simulink model "Improved_Network_Model"  (R2023b)
settings: Solver=FixedStepAuto  StartTime=0.0  StopTime=0.25  FixedStep=h  RelTol=1e-3
values from neighbouring files (symbols this model uses):
  C2 = [ ... (first row only)    [Improved_Network_Constants.m]
  C3 = [ ... (first row only)    [Improved_Network_Constants.m]
  E_e = 0    [Improved_Network_Constants.m]    (also in LIF_Neuron_Constants.m)
  E_i = -70    [Improved_Network_Constants.m]    (also in LIF_Neuron_Constants.m)
  g_lut = g(lut_indices)*1000    [Improved_Network_Constants.m]    (also in LIF_Neuron_Constants.m)
  g_perceptron = 30    [Improved_Network_Constants.m]
  h = 0.0001    [Improved_Network_Constants.m]    (also in LIF_Neuron_Constants.m)
  Rm = 20*10^-2    (= 0.2)    [Improved_Network_Constants.m]    (also in LIF_Neuron_Constants.m)
  tao_m = 50*10^-3    (= 0.05)    [Improved_Network_Constants.m]    (also in LIF_Neuron_Constants.m)
  thr_val = 0.025*1000    (= 25)    [Improved_Network_Constants.m]
  V_thr = -50    [Improved_Network_Constants.m]    (also in LIF_Neuron_Constants.m)
  Vo = -65    [Improved_Network_Constants.m]    (also in LIF_Neuron_Constants.m)
libraries: hdlsllib x168
(part 1 of 4)
settings Model: Creator=Sertan  LastModifiedBy=Sertan
settings OptimizationCC: BlockReduction=off  ConditionallyExecuteInputs=off

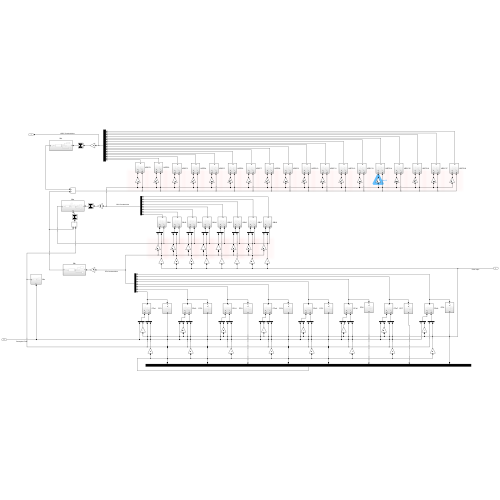
[thumbnail: Simulink's stored preview of the top-level diagram]
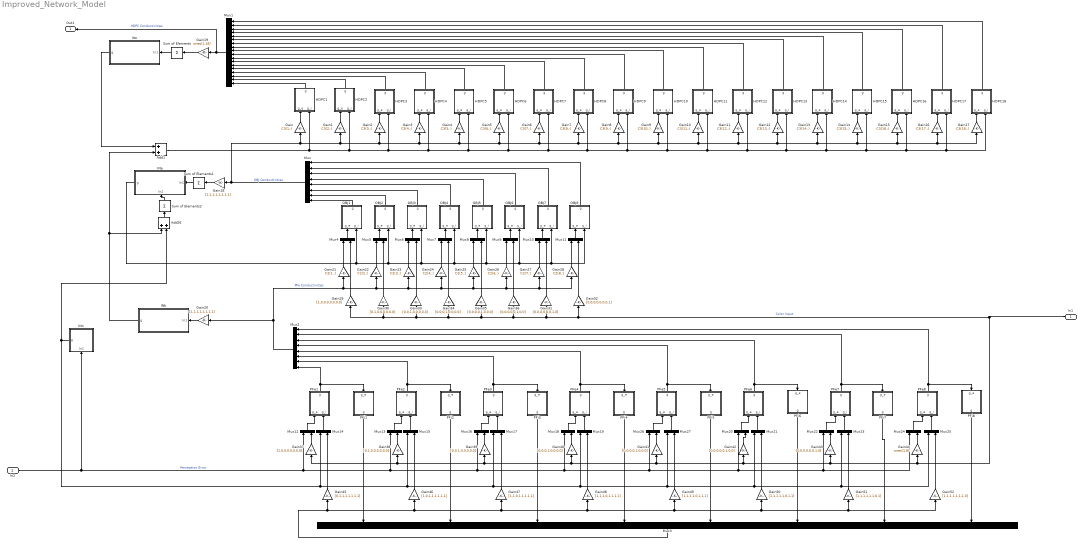
== system Improved_Network_Model ==
  In1 : Inport
  In2 : Inport  Port=2
  Add1 : Sum
  Add26 : Sum
  Gain : Gain  Gain=C3(1,:)
  Gain1 : Gain  Gain=C3(2,:)
  Gain10 : Gain  Gain=C3(11,:)
  Gain11 : Gain  Gain=C3(12,:)
  Gain12 : Gain  Gain=C3(13,:)
  Gain13 : Gain  Gain=C3(14,:)
  Gain14 : Gain  Gain=C3(15,:)
  Gain15 : Gain  Gain=C3(16,:)
  Gain16 : Gain  Gain=C3(17,:)
  Gain17 : Gain  Gain=C3(18,:)
  Gain18 : Gain  Gain=[1,1,1,1,1,1,1,1]
  Gain19 : Gain  Gain=ones(1,18)
  Gain2 : Gain  Gain=C3(3,:)
  Gain20 : Gain  Gain=[1,1,1,1,1,1,1,1]
  Gain21 : Gain  Gain=C2(1,:)  OutDataTypeStr=fixdt(1,16,8)
  Gain22 : Gain  Gain=C2(2,:)  OutDataTypeStr=fixdt(1,16,8)
  Gain23 : Gain  Gain=C2(3,:)  OutDataTypeStr=fixdt(1,16,8)
  Gain24 : Gain  Gain=C2(4,:)  OutDataTypeStr=fixdt(1,16,8)
  Gain25 : Gain  Gain=C2(5,:)  OutDataTypeStr=fixdt(1,16,8)
  Gain26 : Gain  Gain=C2(6,:)  OutDataTypeStr=fixdt(1,16,8)
  Gain27 : Gain  Gain=C2(7,:)  OutDataTypeStr=fixdt(1,16,8)
  Gain28 : Gain  Gain=C2(8,:)  OutDataTypeStr=fixdt(1,16,8)
  Gain29 : Gain  Gain=[1,0,0,0,0,0,0,0]  OutDataTypeStr=fixdt(1,16,8)
  Gain3 : Gain  Gain=C3(4,:)
  Gain30 : Gain  Gain=[0,1,0,0,0,0,0,0]  OutDataTypeStr=fixdt(1,16,8)
  Gain31 : Gain  Gain=[0,0,0,0,0,0,1,0]  OutDataTypeStr=fixdt(1,16,8)
  Gain32 : Gain  Gain=[0,0,0,0,0,0,0,1]  OutDataTypeStr=fixdt(1,16,8)
  Gain33 : Gain  Gain=[0,0,1,0,0,0,0,0]  OutDataTypeStr=fixdt(1,16,8)
  Gain34 : Gain  Gain=[0,0,0,1,0,0,0,0]  OutDataTypeStr=fixdt(1,16,8)
  Gain35 : Gain  Gain=[0,0,0,0,1,0,0,0]  OutDataTypeStr=fixdt(1,16,8)
  Gain36 : Gain  Gain=[0,0,0,0,0,1,0,0]  OutDataTypeStr=fixdt(1,16,8)
  Gain37 : Gain  Gain=[1,0,0,0,0,0,0,0]  OutDataTypeStr=fixdt(1,16,8)
  Gain38 : Gain  Gain=[0,1,0,0,0,0,0,0]  OutDataTypeStr=fixdt(1,16,8)
  Gain39 : Gain  Gain=[0,0,1,0,0,0,0,0]  OutDataTypeStr=fixdt(1,16,8)
  Gain4 : Gain  Gain=C3(5,:)
  Gain40 : Gain  Gain=[0,0,0,1,0,0,0,0]  OutDataTypeStr=fixdt(1,16,8)
  Gain41 : Gain  Gain=[0,0,0,0,1,0,0,0]  OutDataTypeStr=fixdt(1,16,8)
  Gain42 : Gain  Gain=[0,0,0,0,0,1,0,0]  OutDataTypeStr=fixdt(1,16,8)
  Gain43 : Gain  Gain=[0,0,0,0,0,0,1,0]  ParamDataTypeStr=fixdt(1,32,16)  OutDataTypeStr=fixdt(1,16,8)
  Gain44 : Gain  Gain=ones(1,8)  OutDataTypeStr=fixdt(1,16,8)
  Gain45 : Gain  Gain=[0,1,1,1,1,1,1,1]  OutDataTypeStr=fixdt(1,16,8)
  Gain46 : Gain  Gain=[1,0,1,1,1,1,1,1]  OutDataTypeStr=fixdt(1,16,8)
  Gain47 : Gain  Gain=[1,1,0,1,1,1,1,1]  OutDataTypeStr=fixdt(1,16,8)
  Gain48 : Gain  Gain=[1,1,1,0,1,1,1,1]  OutDataTypeStr=fixdt(1,16,8)
  Gain49 : Gain  Gain=[1,1,1,1,0,1,1,1]  OutDataTypeStr=fixdt(1,16,8)
  Gain5 : Gain  Gain=C3(6,:)
  Gain50 : Gain  Gain=[1,1,1,1,1,0,1,1]  OutDataTypeStr=fixdt(1,16,8)
  Gain51 : Gain  Gain=[1,1,1,1,1,1,0,1]  OutDataTypeStr=fixdt(1,16,8)
  Gain52 : Gain  Gain=[1,1,1,1,1,1,1,0]  OutDataTypeStr=fixdt(1,16,8)
  Gain6 : Gain  Gain=C3(7,:)
  Gain7 : Gain  Gain=C3(8,:)
  Gain8 : Gain  Gain=C3(9,:)
  Gain9 : Gain  Gain=C3(10,:)
  HDPC1 : Subsystem
  HDPC10 : Subsystem
  HDPC11 : Subsystem
  HDPC12 : Subsystem
  HDPC13 : Subsystem
  HDPC14 : Subsystem
  HDPC15 : Subsystem
  HDPC16 : Subsystem
  HDPC17 : Subsystem
  HDPC18 : Subsystem
  HDPC2 : Subsystem
  HDPC3 : Subsystem
  HDPC4 : Subsystem
  HDPC5 : Subsystem
  HDPC6 : Subsystem
  HDPC7 : Subsystem
  HDPC8 : Subsystem
  HDPC9 : Subsystem
  INa : Subsystem
      settings: PortSchema="{\"entries\":[{\"content\":{\"sides\":[{\"content\":{\"connectorIds\":[\"In1\"]},\"type\":\"ConnectorPlacement.EquallySpacedRectSide\",\"uuid\":\"7e874ced-1574-4e6e-b75d-ef8740d97bf8\"},{\"content\":{\"connectorIds\":[\"Out1\"],\"side\":\"RIGHT\"},\"type\":\"ConnectorPlacement.EquallySpacedRectSide\",\"uuid\":\"781db9f9-39a3-4cb8-9a9c-5cad13acfbb4\"},{\"content\":{\"side\":\"TOP\"},\"type\":\"ConnectorPlacement.EquallySpacedRectSide\",\"uuid\":\"b182c645-5fec-4e91-86bd-624479001a7a\"},{\"content\":{\"connectorIds\":[\"In2\"],\"side\":\"BOTTOM\"},\"type\":\"ConnectorPlacement.EquallySpacedRectSide\",\"uuid\":\"c39e55bf-3b54-49b1-917e-db485b5d9212\"}]},\"type\":\"ConnectorPlacement.EquallySpacedConnector\",\"uuid\":\"f02879f8-0057-4ea9-bcb0-772f9141270a\"}],\"packageUris\":[\"http://schema.mathworks.com/mf0/Connector/R2020b\"],\"version\":\"1.0\"}"
  INb : Subsystem
  INc : Subsystem
  INn : Subsystem
      settings: PortSchema="{\"entries\":[{\"content\":{\"sides\":[{\"content\":{\"connectorIds\":[\"In1\"]},\"type\":\"ConnectorPlacement.EquallySpacedRectSide\",\"uuid\":\"16d38d29-5ee4-46f0-892f-65d89b640e16\"},{\"content\":{\"side\":\"RIGHT\"},\"type\":\"ConnectorPlacement.EquallySpacedRectSide\",\"uuid\":\"2f107388-f164-4d1d-afe7-0d6d6d47ba29\"},{\"content\":{\"connectorIds\":[\"Out1\"],\"side\":\"TOP\"},\"type\":\"ConnectorPlacement.EquallySpacedRectSide\",\"uuid\":\"02c06e1d-6f05-4188-9ebd-2b49cc778128\"}]},\"type\":\"ConnectorPlacement.EquallySpacedConnector\",\"uuid\":\"ccc7dd7f-c11f-40be-8119-2d95a0a91fe7\"}],\"packageUris\":[\"http://schema.mathworks.com/mf0/Connector/R2020b\"],\"version\":\"1.0\"}"
  Mux : Mux  Inputs=8
  Mux1 : Mux  Inputs=18
  Mux{4..27} (24 alike) : Mux  Inputs=2
  Mux2 : Mux  Inputs=8
  Mux3 : Mux  Inputs=8
  OBJ1 : Subsystem
  OBJ2 : Subsystem
  OBJ3 : Subsystem
  OBJ4 : Subsystem
  OBJ5 : Subsystem
  OBJ6 : Subsystem
  OBJ7 : Subsystem
  OBJ8 : Subsystem
  PFe1 : Subsystem
  PFe2 : Subsystem
  PFe3 : Subsystem
  PFe4 : Subsystem
  PFe5 : Subsystem
  PFe6 : Subsystem
  PFe7 : Subsystem
  PFe8 : Subsystem
  PFi1 : Subsystem
  PFi2 : Subsystem
  PFi3 : Subsystem
  PFi4 : Subsystem
  PFi5 : Subsystem
  PFi6 : Subsystem
  PFi7 : Subsystem
  PFi8 : Subsystem
  Sum of Elements : Sum  Inputs=+
  Sum of Elements1 : Sum  Inputs=+
  Sum of Elements2 : Sum  Inputs=+
  Out1 : Outport  VectorParamsAs1DForOutWhenUnconnected=off
  wires:
  PFe1/1(g) -> PFi1/1(g_e), Mux2/8
  Gain5/1 -> HDPC6/1(g_e)
  Gain33/1 -> Mux6/2
  Gain44/1 -> Mux24/2
  Gain21/1 -> Mux4/1
  Gain/1 -> HDPC1/1(g_e)
  Gain31/1 -> Mux10/2
  PFi7/1(g) -> Mux3/7
  Gain29/1 -> Mux4/2
  Gain20/1 -> INb/1(In1)
  Mux21/1 -> PFe6/2(g_i)
  Gain23/1 -> Mux6/1
  Add26/1 -> Sum of Elements2/1
  HDPC6/1(g) -> Mux1/13
  Mux20/1 -> PFe6/1(g_e)
  Gain7/1 -> HDPC8/1(g_e)
  Mux24/1 -> PFe8/1(g_e)
  Gain6/1 -> HDPC7/1(g_e)
  Gain34/1 -> Mux7/2
  Gain39/1 -> Mux16/2
  Gain42/1 -> Mux20/2
  HDPC14/1(g) -> Mux1/5
  HDPC8/1(g) -> Mux1/11
  Sum of Elements/1 -> INc/1(In1)
  Mux5/1 -> OBJ2/1(g_e)
  Gain27/1 -> Mux10/1
  HDPC17/1(g) -> Mux1/2
  Gain46/1 -> Mux15/2
  Mux13/1 -> PFe2/1(g_e)
  Gain24/1 -> Mux7/1
  Gain32/1 -> Mux11/2
  Mux19/1 -> PFe4/2(g_i)
  Gain19/1 -> Sum of Elements/1
  Gain3/1 -> HDPC4/1(g_e)
  Gain35/1 -> Mux8/2
  Gain47/1 -> Mux17/2
  PFi2/1(g) -> Mux3/2
  HDPC1/1(g) -> Mux1/18
  HDPC4/1(g) -> Mux1/15
  PFi6/1(g) -> Mux3/6
  Mux14/1 -> PFe1/2(g_i)
  Gain18/1 -> Sum of Elements1/1
  HDPC18/1(g) -> Mux1/1
  Gain12/1 -> HDPC13/1(g_e)
  PFe4/1(g) -> PFi4/1(g_e), Mux2/5
  Mux25/1 -> PFe8/2(g_i)
  Mux10/1 -> OBJ7/1(g_e)
  Gain15/1 -> HDPC16/1(g_e)
  Gain28/1 -> Mux11/1
  PFi3/1(g) -> Mux3/3
  INb/1(g) -> Add1/2, Add26/1
  Gain41/1 -> Mux26/2
  Mux12/1 -> PFe1/1(g_e)
  PFe7/1(g) -> PFi7/1(g_e), Mux2/2
  PFe6/1(g) -> PFi6/1(g_e), Mux2/3
  Gain4/1 -> HDPC5/1(g_e)
  PFe8/1(g) -> PFi8/1(g_e), Mux2/1
  Gain49/1 -> Mux27/2
  Gain8/1 -> HDPC9/1(g_e)
  Mux4/1 -> OBJ1/1(g_e)
  HDPC5/1(g) -> Mux1/14
  OBJ1/1(g) -> Mux/8
  PFe3/1(g) -> PFi3/1(g_e), Mux2/6
  Mux23/1 -> PFe7/2(g_i)
  In1/1 -> Gain44/1, Gain43/1, Gain41/1, Gain37/1, Gain38/1, Gain39/1, Gain40/1, Gain42/1, Gain32/1, Gain31/1, Gain36/1, Gain29/1, Gain30/1, Gain33/1, Gain34/1, Gain35/1  "Color Input"
  Gain43/1 -> Mux22/2
  Mux/1 -> Gain18/1, Gain/1, Gain1/1, Gain2/1, Gain5/1, Gain6/1, Gain7/1, Gain9/1, Gain10/1, Gain11/1, Gain12/1, Gain13/1, Gain14/1, Gain15/1, Gain16/1, Gain17/1, Gain8/1, Gain4/1, Gain3/1  "OBJ Conductivities"
  Gain45/1 -> Mux14/2
  OBJ8/1(g) -> Mux/1
  Gain10/1 -> HDPC11/1(g_e)
  PFe5/1(g) -> PFi5/1(g_e), Mux2/4
  PFi8/1(g) -> Mux3/8
  Gain14/1 -> HDPC15/1(g_e)
  Mux9/1 -> OBJ6/1(g_e)
  PFi4/1(g) -> Mux3/4
  Mux16/1 -> PFe3/1(g_e)
  HDPC7/1(g) -> Mux1/12
  Gain13/1 -> HDPC14/1(g_e)
  INa/1(g) -> OBJ1/2(g_i), OBJ2/2(g_i), OBJ3/2(g_i), OBJ4/2(g_i), OBJ5/2(g_i), OBJ6/2(g_i), OBJ8/2(g_i), OBJ7/2(g_i)
  HDPC16/1(g) -> Mux1/3
  Mux11/1 -> OBJ8/1(g_e)
  HDPC2/1(g) -> Mux1/17
  PFe2/1(g) -> PFi2/1(g_e), Mux2/7
  Gain40/1 -> Mux18/2
  Gain9/1 -> HDPC10/1(g_e)
  HDPC9/1(g) -> Mux1/10
  Gain17/1 -> HDPC18/1(g_e)
  Gain1/1 -> HDPC2/1(g_e)
  Gain50/1 -> Mux21/2
  Mux17/1 -> PFe3/2(g_i)
  Sum of Elements2/1 -> INa/2(In2)
  Gain25/1 -> Mux8/1
  HDPC15/1(g) -> Mux1/4
  Mux26/1 -> PFe5/1(g_e)
  Mux15/1 -> PFe2/2(g_i)
  HDPC3/1(g) -> Mux1/16
  Mux22/1 -> PFe7/1(g_e)
  OBJ5/1(g) -> Mux/4
  Gain36/1 -> Mux9/2
  HDPC12/1(g) -> Mux1/7
  Gain30/1 -> Mux5/2
  Gain37/1 -> Mux12/2
  OBJ3/1(g) -> Mux/6
  Mux18/1 -> PFe4/1(g_e)
  OBJ4/1(g) -> Mux/5
  HDPC11/1(g) -> Mux1/8
  OBJ2/1(g) -> Mux/7
  Mux2/1 -> Gain27/1, Gain28/1, Gain26/1, Gain25/1, Gain24/1, Gain23/1, Gain22/1, Gain21/1, Gain20/1  "PFe Conductivities"
  Mux27/1 -> PFe5/2(g_i)
  Gain48/1 -> Mux19/2
  Gain38/1 -> Mux13/2
  Mux7/1 -> OBJ4/1(g_e)
  Gain22/1 -> Mux5/1
  Mux1/1 -> Out1/1, Gain19/1  "HDPC Conductivities"
  Gain11/1 -> HDPC12/1(g_e)
  Mux8/1 -> OBJ5/1(g_e)
  Gain2/1 -> HDPC3/1(g_e)
  Gain16/1 -> HDPC17/1(g_e)
  PFi1/1(g) -> Mux3/1
  In2/1 -> Mux18/1, Mux24/1, Mux22/1, Mux20/1, Mux26/1, Mux16/1, Mux13/1, Mux12/1, INn/1(In1)  "Perception Error"
  Sum of Elements1/1 -> INa/1(In1)
  HDPC13/1(g) -> Mux1/6
  HDPC10/1(g) -> Mux1/9
  Gain51/1 -> Mux23/2
  Mux3/1 -> Gain52/1, Gain51/1, Gain50/1, Gain49/1, Gain48/1, Gain47/1, Gain46/1, Gain45/1
  Mux6/1 -> OBJ3/1(g_e)
  PFi5/1(g) -> Mux3/5
  Gain52/1 -> Mux25/2
  INn/1(g) -> Add26/2, Mux25/1, Mux23/1, Mux21/1, Mux27/1, Mux19/1, Mux17/1, Mux15/1, Mux14/1
  Gain26/1 -> Mux9/1
  INc/1(g) -> Add1/1
  OBJ7/1(g) -> Mux/2
  Add1/1 -> HDPC1/2(g_i), HDPC2/2(g_i), HDPC3/2(g_i), HDPC4/2(g_i), HDPC5/2(g_i), HDPC6/2(g_i), HDPC7/2(g_i), HDPC8/2(g_i), HDPC9/2(g_i), HDPC10/2(g_i), HDPC11/2(g_i), HDPC12/2(g_i), HDPC13/2(g_i), HDPC14/2(g_i), HDPC15/2(g_i), HDPC16/2(g_i), HDPC17/2(g_i), HDPC18/2(g_i)
  OBJ6/1(g) -> Mux/3

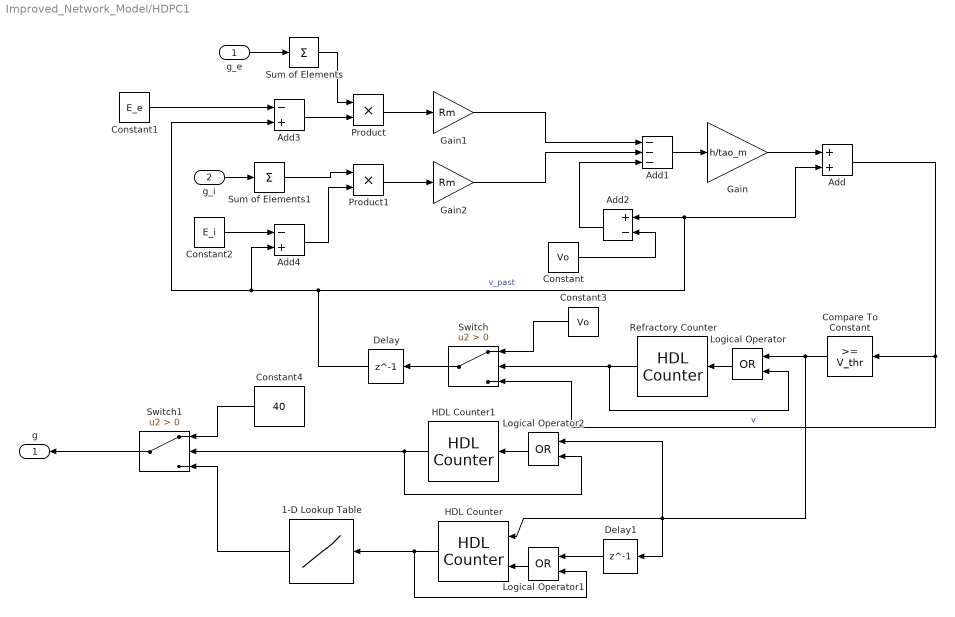
== system Improved_Network_Model/HDPC1 ==
  g_e : Inport
  g_i : Inport  Port=2
  1-D Lookup Table : Lookup_n-D  NumberOfTableDimensions=1  LookupTableObject=''  BreakpointsForDimension1=[0:201]  BreakpointsForDimension1FirstPoint=10  BreakpointsForDimension2FirstPoint=10  BreakpointsForDimension1Spacing=12  BreakpointsForDimension2Spacing=12  BreakpointsForDimension1DataTypeStr=Inherit: Inherit from 'Breakpoint data'  IndexSearchMethod=Evenly spaced points  Table=g_lut  InterpMethod=Flat  DiagnosticForOutOfRangeInput=Error  InternalRulePriority=Speed  OutDataTypeStr=fixdt(1,16,8)  RndMeth=Simplest
  Add : Sum
  Add1 : Sum  Inputs=---
  Add2 : Sum  Inputs=+-
  Add3 : Sum  Inputs=-+
  Add4 : Sum  Inputs=-+
  Compare To Constant : hdlsllib/Logic and Bit Operations/Compare To Constant  relop=>=  const=V_thr  OutDataTypeStr=boolean
  Constant : Constant  Value=Vo  OutDataTypeStr=fixdt(1,16,8)
  Constant1 : Constant  Value=E_e  OutDataTypeStr=fixdt(1,16,8)
  Constant2 : Constant  Value=E_i  OutDataTypeStr=fixdt(1,16,8)
  Constant3 : Constant  Value=Vo  OutDataTypeStr=fixdt(1,16,8)
  Constant4 : Constant  Value=40  OutDataTypeStr=fixdt(1,16,8)
  Delay : Delay  DelayLength=1  InitialCondition=Vo
  Delay1 : Delay  DelayLength=1  InitialCondition=0
  Gain : Gain  Gain=h/tao_m  OutDataTypeStr=fixdt(1,16,8)
  Gain1 : Gain  Gain=Rm
  Gain2 : Gain  Gain=Rm
  HDL Counter : hdlsllib/Sources/HDL Counter  CountType=Count limited  CountInit=0  CountStep=1  CountMax=length(g_lut)-1  CountFromType=Initial value  CountFrom=0  CountResetPort=on  CountLoadPort=off  CountEnbPort=on  CountDirPort=off  CountHitOutputPort=off  CountDataType=Unsigned  CountWordLen=8  CountFracLen=0  CountSampTime=1
  HDL Counter1 : hdlsllib/Sources/HDL Counter  CountType=Count limited  CountInit=0  CountStep=1  CountMax=2  CountFromType=Initial value  CountFrom=0  CountResetPort=off  CountLoadPort=off  CountEnbPort=on  CountDirPort=off  CountHitOutputPort=off  CountDataType=Unsigned  CountWordLen=8  CountFracLen=0  CountSampTime=1
  Logical Operator : Logic  Operator=OR  AllPortsSameDT=off  OutDataTypeStr=boolean
  Logical Operator1 : Logic  Operator=OR  AllPortsSameDT=off  OutDataTypeStr=boolean
  Logical Operator2 : Logic  Operator=OR  AllPortsSameDT=off  OutDataTypeStr=boolean
  Product : Product
  Product1 : Product
  Refractory Counter : hdlsllib/Sources/HDL Counter  CountType=Count limited  CountInit=0  CountStep=1  CountMax=r_time  CountFromType=Initial value  CountFrom=0  CountResetPort=off  CountLoadPort=off  CountEnbPort=on  CountDirPort=off  CountHitOutputPort=off  CountDataType=Unsigned  CountWordLen=8  CountFracLen=0  CountSampTime=1
  Sum of Elements : Sum  Inputs=+
  Sum of Elements1 : Sum  Inputs=+
  Switch : Switch  Criteria=u2 > Threshold  SaturateOnIntegerOverflow=off  InputSameDT=off
  Switch1 : Switch  Criteria=u2 > Threshold  OutDataTypeStr=fixdt(1,16,8)  SaturateOnIntegerOverflow=off  InputSameDT=off
  g : Outport  VectorParamsAs1DForOutWhenUnconnected=off
  wires:
  Constant/1 -> Add2/2
  Delay/1 -> Add3/2, Add4/2, Add/2, Add2/1  "v_past"
  Add/1 -> Switch/3, Compare To Constant/1  "v"
  g_i/1 -> Sum of Elements1/1
  Gain1/1 -> Add1/1
  Add2/1 -> Add1/3
  Add1/1 -> Gain/1
  Add4/1 -> Product1/2
  Product/1 -> Gain1/1
  Add3/1 -> Product/2
  Gain2/1 -> Add1/2
  Gain/1 -> Add/1
  Sum of Elements/1 -> Product/1
  Constant1/1 -> Add3/1
  Constant2/1 -> Add4/1
  Product1/1 -> Gain2/1
  Constant3/1 -> Switch/1
  Refractory Counter/1 -> Logical Operator/2, Switch/2
  Logical Operator/1 -> Refractory Counter/1
  HDL Counter/1 -> Logical Operator1/2, 1-D Lookup Table/1
  Switch1/1 -> g/1
  Switch/1 -> Delay/1
  1-D Lookup Table/1 -> Switch1/3
  Logical Operator1/1 -> HDL Counter/2
  Delay1/1 -> Logical Operator1/1
  Constant4/1 -> Switch1/1
  Logical Operator2/1 -> HDL Counter1/1
  HDL Counter1/1 -> Switch1/2, Logical Operator2/2
  Compare To Constant/1 -> Logical Operator/1, Delay1/1, Logical Operator2/1, HDL Counter/1
  g_e/1 -> Sum of Elements/1
  Sum of Elements1/1 -> Product1/1

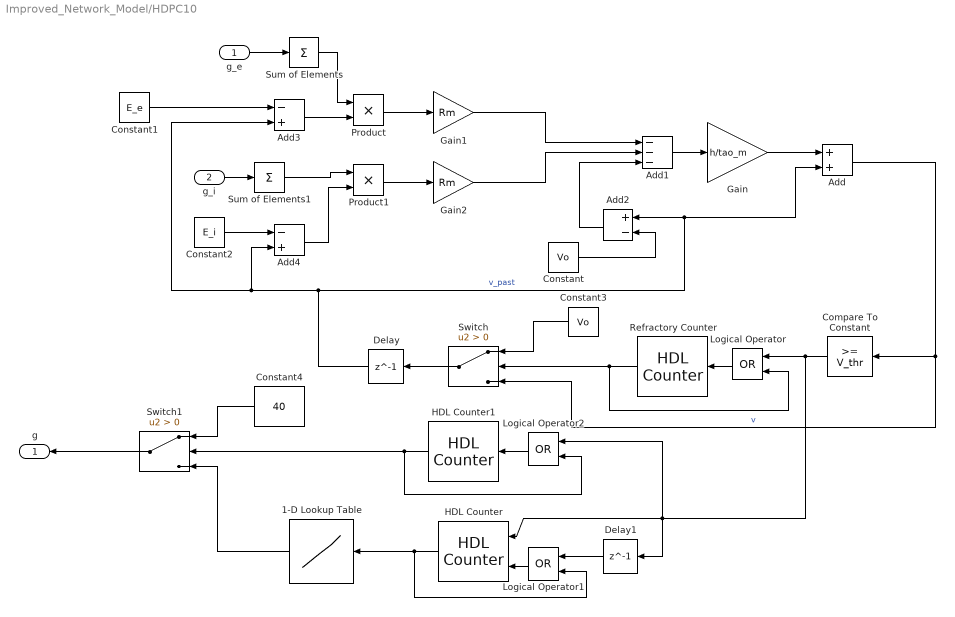
== system Improved_Network_Model/HDPC10 ==
  g_e : Inport
  g_i : Inport  Port=2
  1-D Lookup Table : Lookup_n-D  NumberOfTableDimensions=1  LookupTableObject=''  BreakpointsForDimension1=[0:201]  BreakpointsForDimension1FirstPoint=10  BreakpointsForDimension2FirstPoint=10  BreakpointsForDimension1Spacing=12  BreakpointsForDimension2Spacing=12  BreakpointsForDimension1DataTypeStr=Inherit: Inherit from 'Breakpoint data'  IndexSearchMethod=Evenly spaced points  Table=g_lut  InterpMethod=Flat  DiagnosticForOutOfRangeInput=Error  InternalRulePriority=Speed  OutDataTypeStr=fixdt(1,16,8)  RndMeth=Simplest
  Add : Sum
  Add1 : Sum  Inputs=---
  Add2 : Sum  Inputs=+-
  Add3 : Sum  Inputs=-+
  Add4 : Sum  Inputs=-+
  Compare To Constant : hdlsllib/Logic and Bit Operations/Compare To Constant  relop=>=  const=V_thr  OutDataTypeStr=boolean
  Constant : Constant  Value=Vo  OutDataTypeStr=fixdt(1,16,8)
  Constant1 : Constant  Value=E_e  OutDataTypeStr=fixdt(1,16,8)
  Constant2 : Constant  Value=E_i  OutDataTypeStr=fixdt(1,16,8)
  Constant3 : Constant  Value=Vo  OutDataTypeStr=fixdt(1,16,8)
  Constant4 : Constant  Value=40  OutDataTypeStr=fixdt(1,16,8)
  Delay : Delay  DelayLength=1  InitialCondition=Vo
  Delay1 : Delay  DelayLength=1  InitialCondition=0
  Gain : Gain  Gain=h/tao_m  OutDataTypeStr=fixdt(1,16,8)
  Gain1 : Gain  Gain=Rm
  Gain2 : Gain  Gain=Rm
  HDL Counter : hdlsllib/Sources/HDL Counter  CountType=Count limited  CountInit=0  CountStep=1  CountMax=length(g_lut)-1  CountFromType=Initial value  CountFrom=0  CountResetPort=on  CountLoadPort=off  CountEnbPort=on  CountDirPort=off  CountHitOutputPort=off  CountDataType=Unsigned  CountWordLen=8  CountFracLen=0  CountSampTime=1
  HDL Counter1 : hdlsllib/Sources/HDL Counter  CountType=Count limited  CountInit=0  CountStep=1  CountMax=2  CountFromType=Initial value  CountFrom=0  CountResetPort=off  CountLoadPort=off  CountEnbPort=on  CountDirPort=off  CountHitOutputPort=off  CountDataType=Unsigned  CountWordLen=8  CountFracLen=0  CountSampTime=1
  Logical Operator : Logic  Operator=OR  AllPortsSameDT=off  OutDataTypeStr=boolean
  Logical Operator1 : Logic  Operator=OR  AllPortsSameDT=off  OutDataTypeStr=boolean
  Logical Operator2 : Logic  Operator=OR  AllPortsSameDT=off  OutDataTypeStr=boolean
  Product : Product
  Product1 : Product
  Refractory Counter : hdlsllib/Sources/HDL Counter  CountType=Count limited  CountInit=0  CountStep=1  CountMax=r_time  CountFromType=Initial value  CountFrom=0  CountResetPort=off  CountLoadPort=off  CountEnbPort=on  CountDirPort=off  CountHitOutputPort=off  CountDataType=Unsigned  CountWordLen=8  CountFracLen=0  CountSampTime=1
  Sum of Elements : Sum  Inputs=+
  Sum of Elements1 : Sum  Inputs=+
  Switch : Switch  Criteria=u2 > Threshold  SaturateOnIntegerOverflow=off  InputSameDT=off
  Switch1 : Switch  Criteria=u2 > Threshold  OutDataTypeStr=fixdt(1,16,8)  SaturateOnIntegerOverflow=off  InputSameDT=off
  g : Outport  VectorParamsAs1DForOutWhenUnconnected=off
  wires:
  Constant/1 -> Add2/2
  Delay/1 -> Add3/2, Add4/2, Add/2, Add2/1  "v_past"
  Add/1 -> Switch/3, Compare To Constant/1  "v"
  g_i/1 -> Sum of Elements1/1
  Gain1/1 -> Add1/1
  Add2/1 -> Add1/3
  Add1/1 -> Gain/1
  Add4/1 -> Product1/2
  Product/1 -> Gain1/1
  Add3/1 -> Product/2
  Gain2/1 -> Add1/2
  Gain/1 -> Add/1
  Sum of Elements/1 -> Product/1
  Constant1/1 -> Add3/1
  Constant2/1 -> Add4/1
  Product1/1 -> Gain2/1
  Constant3/1 -> Switch/1
  Refractory Counter/1 -> Logical Operator/2, Switch/2
  Logical Operator/1 -> Refractory Counter/1
  HDL Counter/1 -> Logical Operator1/2, 1-D Lookup Table/1
  Switch1/1 -> g/1
  Switch/1 -> Delay/1
  1-D Lookup Table/1 -> Switch1/3
  Logical Operator1/1 -> HDL Counter/2
  Delay1/1 -> Logical Operator1/1
  Constant4/1 -> Switch1/1
  Logical Operator2/1 -> HDL Counter1/1
  HDL Counter1/1 -> Switch1/2, Logical Operator2/2
  Compare To Constant/1 -> Logical Operator/1, Delay1/1, Logical Operator2/1, HDL Counter/1
  g_e/1 -> Sum of Elements/1
  Sum of Elements1/1 -> Product1/1

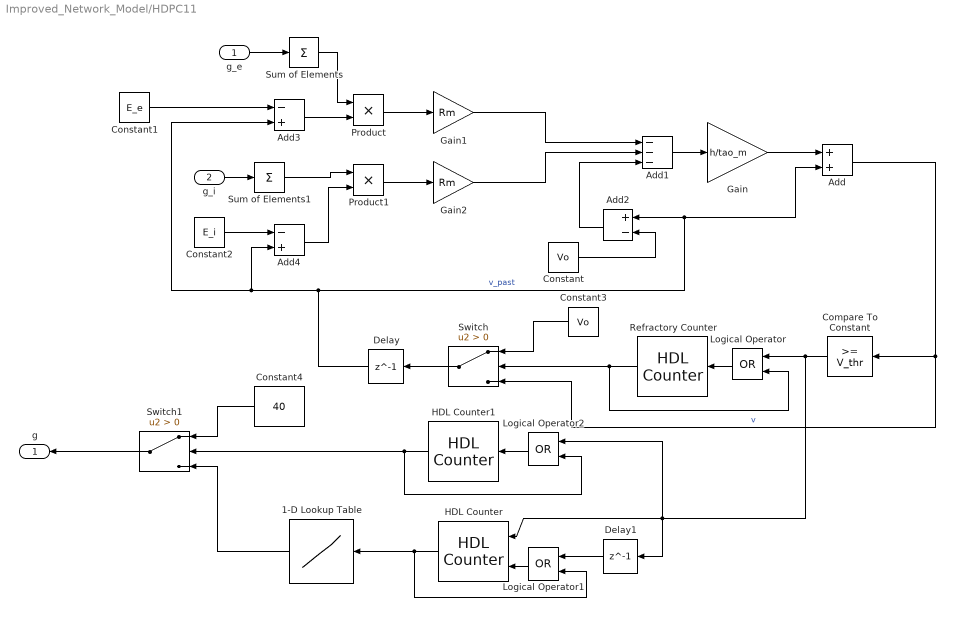
== system Improved_Network_Model/HDPC11 ==
  g_e : Inport
  g_i : Inport  Port=2
  1-D Lookup Table : Lookup_n-D  NumberOfTableDimensions=1  LookupTableObject=''  BreakpointsForDimension1=[0:201]  BreakpointsForDimension1FirstPoint=10  BreakpointsForDimension2FirstPoint=10  BreakpointsForDimension1Spacing=12  BreakpointsForDimension2Spacing=12  BreakpointsForDimension1DataTypeStr=Inherit: Inherit from 'Breakpoint data'  IndexSearchMethod=Evenly spaced points  Table=g_lut  InterpMethod=Flat  DiagnosticForOutOfRangeInput=Error  InternalRulePriority=Speed  OutDataTypeStr=fixdt(1,16,8)  RndMeth=Simplest
  Add : Sum
  Add1 : Sum  Inputs=---
  Add2 : Sum  Inputs=+-
  Add3 : Sum  Inputs=-+
  Add4 : Sum  Inputs=-+
  Compare To Constant : hdlsllib/Logic and Bit Operations/Compare To Constant  relop=>=  const=V_thr  OutDataTypeStr=boolean
  Constant : Constant  Value=Vo  OutDataTypeStr=fixdt(1,16,8)
  Constant1 : Constant  Value=E_e  OutDataTypeStr=fixdt(1,16,8)
  Constant2 : Constant  Value=E_i  OutDataTypeStr=fixdt(1,16,8)
  Constant3 : Constant  Value=Vo  OutDataTypeStr=fixdt(1,16,8)
  Constant4 : Constant  Value=40  OutDataTypeStr=fixdt(1,16,8)
  Delay : Delay  DelayLength=1  InitialCondition=Vo
  Delay1 : Delay  DelayLength=1  InitialCondition=0
  Gain : Gain  Gain=h/tao_m  OutDataTypeStr=fixdt(1,16,8)
  Gain1 : Gain  Gain=Rm
  Gain2 : Gain  Gain=Rm
  HDL Counter : hdlsllib/Sources/HDL Counter  CountType=Count limited  CountInit=0  CountStep=1  CountMax=length(g_lut)-1  CountFromType=Initial value  CountFrom=0  CountResetPort=on  CountLoadPort=off  CountEnbPort=on  CountDirPort=off  CountHitOutputPort=off  CountDataType=Unsigned  CountWordLen=8  CountFracLen=0  CountSampTime=1
  HDL Counter1 : hdlsllib/Sources/HDL Counter  CountType=Count limited  CountInit=0  CountStep=1  CountMax=2  CountFromType=Initial value  CountFrom=0  CountResetPort=off  CountLoadPort=off  CountEnbPort=on  CountDirPort=off  CountHitOutputPort=off  CountDataType=Unsigned  CountWordLen=8  CountFracLen=0  CountSampTime=1
  Logical Operator : Logic  Operator=OR  AllPortsSameDT=off  OutDataTypeStr=boolean
  Logical Operator1 : Logic  Operator=OR  AllPortsSameDT=off  OutDataTypeStr=boolean
  Logical Operator2 : Logic  Operator=OR  AllPortsSameDT=off  OutDataTypeStr=boolean
  Product : Product
  Product1 : Product
  Refractory Counter : hdlsllib/Sources/HDL Counter  CountType=Count limited  CountInit=0  CountStep=1  CountMax=r_time  CountFromType=Initial value  CountFrom=0  CountResetPort=off  CountLoadPort=off  CountEnbPort=on  CountDirPort=off  CountHitOutputPort=off  CountDataType=Unsigned  CountWordLen=8  CountFracLen=0  CountSampTime=1
  Sum of Elements : Sum  Inputs=+
  Sum of Elements1 : Sum  Inputs=+
  Switch : Switch  Criteria=u2 > Threshold  SaturateOnIntegerOverflow=off  InputSameDT=off
  Switch1 : Switch  Criteria=u2 > Threshold  OutDataTypeStr=fixdt(1,16,8)  SaturateOnIntegerOverflow=off  InputSameDT=off
  g : Outport  VectorParamsAs1DForOutWhenUnconnected=off
  wires:
  Constant/1 -> Add2/2
  Delay/1 -> Add3/2, Add4/2, Add/2, Add2/1  "v_past"
  Add/1 -> Switch/3, Compare To Constant/1  "v"
  g_i/1 -> Sum of Elements1/1
  Gain1/1 -> Add1/1
  Add2/1 -> Add1/3
  Add1/1 -> Gain/1
  Add4/1 -> Product1/2
  Product/1 -> Gain1/1
  Add3/1 -> Product/2
  Gain2/1 -> Add1/2
  Gain/1 -> Add/1
  Sum of Elements/1 -> Product/1
  Constant1/1 -> Add3/1
  Constant2/1 -> Add4/1
  Product1/1 -> Gain2/1
  Constant3/1 -> Switch/1
  Refractory Counter/1 -> Logical Operator/2, Switch/2
  Logical Operator/1 -> Refractory Counter/1
  HDL Counter/1 -> Logical Operator1/2, 1-D Lookup Table/1
  Switch1/1 -> g/1
  Switch/1 -> Delay/1
  1-D Lookup Table/1 -> Switch1/3
  Logical Operator1/1 -> HDL Counter/2
  Delay1/1 -> Logical Operator1/1
  Constant4/1 -> Switch1/1
  Logical Operator2/1 -> HDL Counter1/1
  HDL Counter1/1 -> Switch1/2, Logical Operator2/2
  Compare To Constant/1 -> Logical Operator/1, Delay1/1, Logical Operator2/1, HDL Counter/1
  g_e/1 -> Sum of Elements/1
  Sum of Elements1/1 -> Product1/1

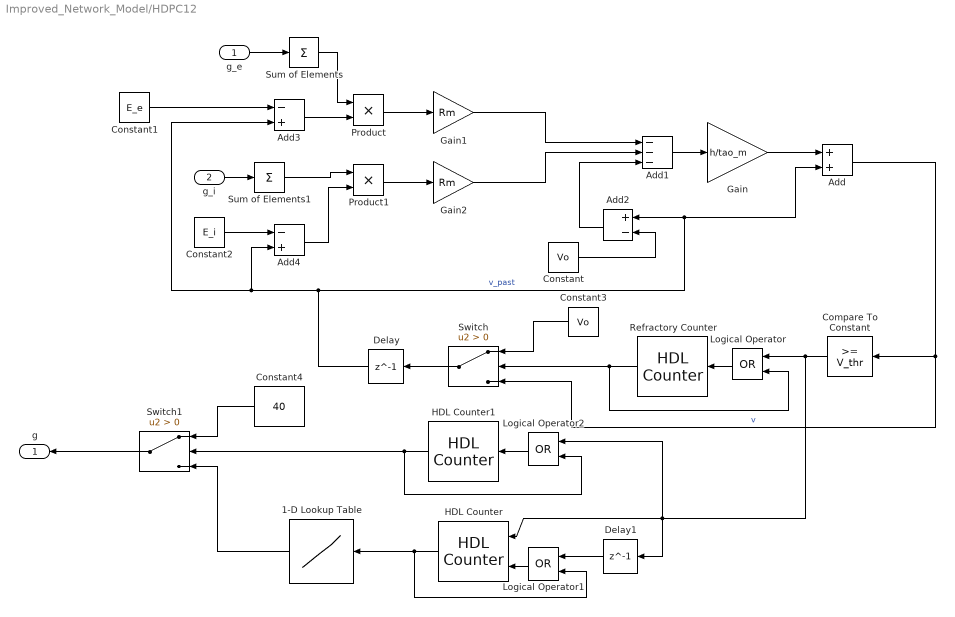
== system Improved_Network_Model/HDPC12 ==
  g_e : Inport
  g_i : Inport  Port=2
  1-D Lookup Table : Lookup_n-D  NumberOfTableDimensions=1  LookupTableObject=''  BreakpointsForDimension1=[0:201]  BreakpointsForDimension1FirstPoint=10  BreakpointsForDimension2FirstPoint=10  BreakpointsForDimension1Spacing=12  BreakpointsForDimension2Spacing=12  BreakpointsForDimension1DataTypeStr=Inherit: Inherit from 'Breakpoint data'  IndexSearchMethod=Evenly spaced points  Table=g_lut  InterpMethod=Flat  DiagnosticForOutOfRangeInput=Error  InternalRulePriority=Speed  OutDataTypeStr=fixdt(1,16,8)  RndMeth=Simplest
  Add : Sum
  Add1 : Sum  Inputs=---
  Add2 : Sum  Inputs=+-
  Add3 : Sum  Inputs=-+
  Add4 : Sum  Inputs=-+
  Compare To Constant : hdlsllib/Logic and Bit Operations/Compare To Constant  relop=>=  const=V_thr  OutDataTypeStr=boolean
  Constant : Constant  Value=Vo  OutDataTypeStr=fixdt(1,16,8)
  Constant1 : Constant  Value=E_e  OutDataTypeStr=fixdt(1,16,8)
  Constant2 : Constant  Value=E_i  OutDataTypeStr=fixdt(1,16,8)
  Constant3 : Constant  Value=Vo  OutDataTypeStr=fixdt(1,16,8)
  Constant4 : Constant  Value=40  OutDataTypeStr=fixdt(1,16,8)
  Delay : Delay  DelayLength=1  InitialCondition=Vo
  Delay1 : Delay  DelayLength=1  InitialCondition=0
  Gain : Gain  Gain=h/tao_m  OutDataTypeStr=fixdt(1,16,8)
  Gain1 : Gain  Gain=Rm
  Gain2 : Gain  Gain=Rm
  HDL Counter : hdlsllib/Sources/HDL Counter  CountType=Count limited  CountInit=0  CountStep=1  CountMax=length(g_lut)-1  CountFromType=Initial value  CountFrom=0  CountResetPort=on  CountLoadPort=off  CountEnbPort=on  CountDirPort=off  CountHitOutputPort=off  CountDataType=Unsigned  CountWordLen=8  CountFracLen=0  CountSampTime=1
  HDL Counter1 : hdlsllib/Sources/HDL Counter  CountType=Count limited  CountInit=0  CountStep=1  CountMax=2  CountFromType=Initial value  CountFrom=0  CountResetPort=off  CountLoadPort=off  CountEnbPort=on  CountDirPort=off  CountHitOutputPort=off  CountDataType=Unsigned  CountWordLen=8  CountFracLen=0  CountSampTime=1
  Logical Operator : Logic  Operator=OR  AllPortsSameDT=off  OutDataTypeStr=boolean
  Logical Operator1 : Logic  Operator=OR  AllPortsSameDT=off  OutDataTypeStr=boolean
  Logical Operator2 : Logic  Operator=OR  AllPortsSameDT=off  OutDataTypeStr=boolean
  Product : Product
  Product1 : Product
  Refractory Counter : hdlsllib/Sources/HDL Counter  CountType=Count limited  CountInit=0  CountStep=1  CountMax=r_time  CountFromType=Initial value  CountFrom=0  CountResetPort=off  CountLoadPort=off  CountEnbPort=on  CountDirPort=off  CountHitOutputPort=off  CountDataType=Unsigned  CountWordLen=8  CountFracLen=0  CountSampTime=1
  Sum of Elements : Sum  Inputs=+
  Sum of Elements1 : Sum  Inputs=+
  Switch : Switch  Criteria=u2 > Threshold  SaturateOnIntegerOverflow=off  InputSameDT=off
  Switch1 : Switch  Criteria=u2 > Threshold  OutDataTypeStr=fixdt(1,16,8)  SaturateOnIntegerOverflow=off  InputSameDT=off
  g : Outport  VectorParamsAs1DForOutWhenUnconnected=off
  wires:
  Constant/1 -> Add2/2
  Delay/1 -> Add3/2, Add4/2, Add/2, Add2/1  "v_past"
  Add/1 -> Switch/3, Compare To Constant/1  "v"
  g_i/1 -> Sum of Elements1/1
  Gain1/1 -> Add1/1
  Add2/1 -> Add1/3
  Add1/1 -> Gain/1
  Add4/1 -> Product1/2
  Product/1 -> Gain1/1
  Add3/1 -> Product/2
  Gain2/1 -> Add1/2
  Gain/1 -> Add/1
  Sum of Elements/1 -> Product/1
  Constant1/1 -> Add3/1
  Constant2/1 -> Add4/1
  Product1/1 -> Gain2/1
  Constant3/1 -> Switch/1
  Refractory Counter/1 -> Logical Operator/2, Switch/2
  Logical Operator/1 -> Refractory Counter/1
  HDL Counter/1 -> Logical Operator1/2, 1-D Lookup Table/1
  Switch1/1 -> g/1
  Switch/1 -> Delay/1
  1-D Lookup Table/1 -> Switch1/3
  Logical Operator1/1 -> HDL Counter/2
  Delay1/1 -> Logical Operator1/1
  Constant4/1 -> Switch1/1
  Logical Operator2/1 -> HDL Counter1/1
  HDL Counter1/1 -> Switch1/2, Logical Operator2/2
  Compare To Constant/1 -> Logical Operator/1, Delay1/1, Logical Operator2/1, HDL Counter/1
  g_e/1 -> Sum of Elements/1
  Sum of Elements1/1 -> Product1/1

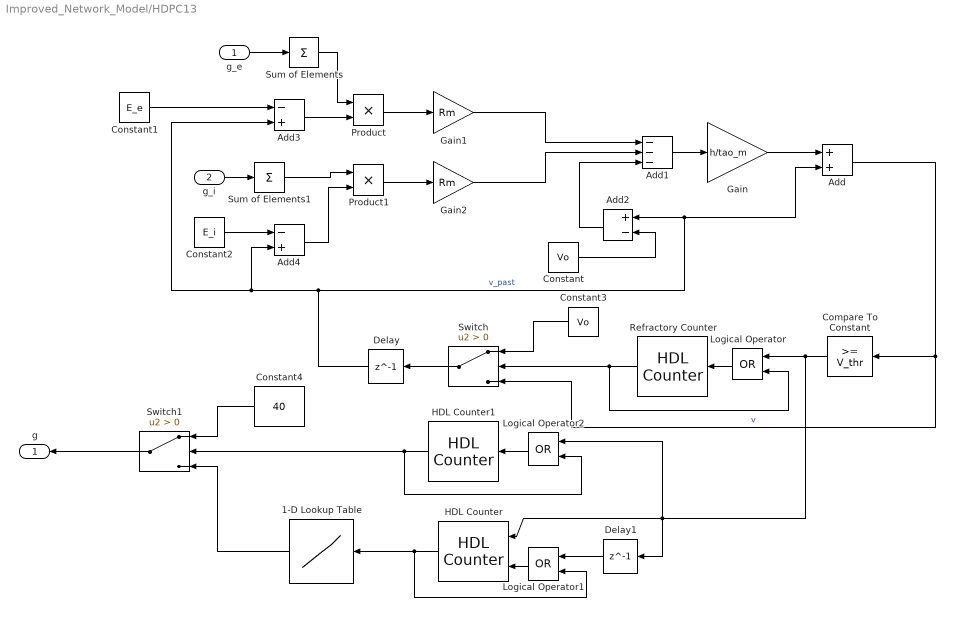
== system Improved_Network_Model/HDPC13 ==
  g_e : Inport
  g_i : Inport  Port=2
  1-D Lookup Table : Lookup_n-D  NumberOfTableDimensions=1  LookupTableObject=''  BreakpointsForDimension1=[0:201]  BreakpointsForDimension1FirstPoint=10  BreakpointsForDimension2FirstPoint=10  BreakpointsForDimension1Spacing=12  BreakpointsForDimension2Spacing=12  BreakpointsForDimension1DataTypeStr=Inherit: Inherit from 'Breakpoint data'  IndexSearchMethod=Evenly spaced points  Table=g_lut  InterpMethod=Flat  DiagnosticForOutOfRangeInput=Error  InternalRulePriority=Speed  OutDataTypeStr=fixdt(1,16,8)  RndMeth=Simplest
  Add : Sum
  Add1 : Sum  Inputs=---
  Add2 : Sum  Inputs=+-
  Add3 : Sum  Inputs=-+
  Add4 : Sum  Inputs=-+
  Compare To Constant : hdlsllib/Logic and Bit Operations/Compare To Constant  relop=>=  const=V_thr  OutDataTypeStr=boolean
  Constant : Constant  Value=Vo  OutDataTypeStr=fixdt(1,16,8)
  Constant1 : Constant  Value=E_e  OutDataTypeStr=fixdt(1,16,8)
  Constant2 : Constant  Value=E_i  OutDataTypeStr=fixdt(1,16,8)
  Constant3 : Constant  Value=Vo  OutDataTypeStr=fixdt(1,16,8)
  Constant4 : Constant  Value=40  OutDataTypeStr=fixdt(1,16,8)
  Delay : Delay  DelayLength=1  InitialCondition=Vo
  Delay1 : Delay  DelayLength=1  InitialCondition=0
  Gain : Gain  Gain=h/tao_m  OutDataTypeStr=fixdt(1,16,8)
  Gain1 : Gain  Gain=Rm
  Gain2 : Gain  Gain=Rm
  HDL Counter : hdlsllib/Sources/HDL Counter  CountType=Count limited  CountInit=0  CountStep=1  CountMax=length(g_lut)-1  CountFromType=Initial value  CountFrom=0  CountResetPort=on  CountLoadPort=off  CountEnbPort=on  CountDirPort=off  CountHitOutputPort=off  CountDataType=Unsigned  CountWordLen=8  CountFracLen=0  CountSampTime=1
  HDL Counter1 : hdlsllib/Sources/HDL Counter  CountType=Count limited  CountInit=0  CountStep=1  CountMax=2  CountFromType=Initial value  CountFrom=0  CountResetPort=off  CountLoadPort=off  CountEnbPort=on  CountDirPort=off  CountHitOutputPort=off  CountDataType=Unsigned  CountWordLen=8  CountFracLen=0  CountSampTime=1
  Logical Operator : Logic  Operator=OR  AllPortsSameDT=off  OutDataTypeStr=boolean
  Logical Operator1 : Logic  Operator=OR  AllPortsSameDT=off  OutDataTypeStr=boolean
  Logical Operator2 : Logic  Operator=OR  AllPortsSameDT=off  OutDataTypeStr=boolean
  Product : Product
  Product1 : Product
  Refractory Counter : hdlsllib/Sources/HDL Counter  CountType=Count limited  CountInit=0  CountStep=1  CountMax=r_time  CountFromType=Initial value  CountFrom=0  CountResetPort=off  CountLoadPort=off  CountEnbPort=on  CountDirPort=off  CountHitOutputPort=off  CountDataType=Unsigned  CountWordLen=8  CountFracLen=0  CountSampTime=1
  Sum of Elements : Sum  Inputs=+
  Sum of Elements1 : Sum  Inputs=+
  Switch : Switch  Criteria=u2 > Threshold  SaturateOnIntegerOverflow=off  InputSameDT=off
  Switch1 : Switch  Criteria=u2 > Threshold  OutDataTypeStr=fixdt(1,16,8)  SaturateOnIntegerOverflow=off  InputSameDT=off
  g : Outport  VectorParamsAs1DForOutWhenUnconnected=off
  wires:
  Constant/1 -> Add2/2
  Delay/1 -> Add3/2, Add4/2, Add/2, Add2/1  "v_past"
  Add/1 -> Switch/3, Compare To Constant/1  "v"
  g_i/1 -> Sum of Elements1/1
  Gain1/1 -> Add1/1
  Add2/1 -> Add1/3
  Add1/1 -> Gain/1
  Add4/1 -> Product1/2
  Product/1 -> Gain1/1
  Add3/1 -> Product/2
  Gain2/1 -> Add1/2
  Gain/1 -> Add/1
  Sum of Elements/1 -> Product/1
  Constant1/1 -> Add3/1
  Constant2/1 -> Add4/1
  Product1/1 -> Gain2/1
  Constant3/1 -> Switch/1
  Refractory Counter/1 -> Logical Operator/2, Switch/2
  Logical Operator/1 -> Refractory Counter/1
  HDL Counter/1 -> Logical Operator1/2, 1-D Lookup Table/1
  Switch1/1 -> g/1
  Switch/1 -> Delay/1
  1-D Lookup Table/1 -> Switch1/3
  Logical Operator1/1 -> HDL Counter/2
  Delay1/1 -> Logical Operator1/1
  Constant4/1 -> Switch1/1
  Logical Operator2/1 -> HDL Counter1/1
  HDL Counter1/1 -> Switch1/2, Logical Operator2/2
  Compare To Constant/1 -> Logical Operator/1, Delay1/1, Logical Operator2/1, HDL Counter/1
  g_e/1 -> Sum of Elements/1
  Sum of Elements1/1 -> Product1/1

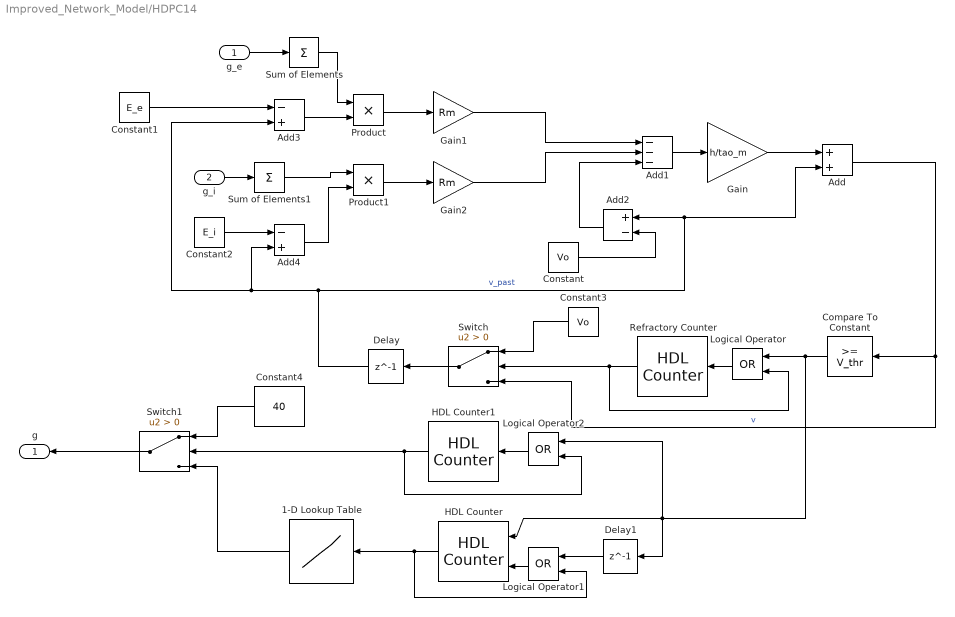
== system Improved_Network_Model/HDPC14 ==
  g_e : Inport
  g_i : Inport  Port=2
  1-D Lookup Table : Lookup_n-D  NumberOfTableDimensions=1  LookupTableObject=''  BreakpointsForDimension1=[0:201]  BreakpointsForDimension1FirstPoint=10  BreakpointsForDimension2FirstPoint=10  BreakpointsForDimension1Spacing=12  BreakpointsForDimension2Spacing=12  BreakpointsForDimension1DataTypeStr=Inherit: Inherit from 'Breakpoint data'  IndexSearchMethod=Evenly spaced points  Table=g_lut  InterpMethod=Flat  DiagnosticForOutOfRangeInput=Error  InternalRulePriority=Speed  OutDataTypeStr=fixdt(1,16,8)  RndMeth=Simplest
  Add : Sum
  Add1 : Sum  Inputs=---
  Add2 : Sum  Inputs=+-
  Add3 : Sum  Inputs=-+
  Add4 : Sum  Inputs=-+
  Compare To Constant : hdlsllib/Logic and Bit Operations/Compare To Constant  relop=>=  const=V_thr  OutDataTypeStr=boolean
  Constant : Constant  Value=Vo  OutDataTypeStr=fixdt(1,16,8)
  Constant1 : Constant  Value=E_e  OutDataTypeStr=fixdt(1,16,8)
  Constant2 : Constant  Value=E_i  OutDataTypeStr=fixdt(1,16,8)
  Constant3 : Constant  Value=Vo  OutDataTypeStr=fixdt(1,16,8)
  Constant4 : Constant  Value=40  OutDataTypeStr=fixdt(1,16,8)
  Delay : Delay  DelayLength=1  InitialCondition=Vo
  Delay1 : Delay  DelayLength=1  InitialCondition=0
  Gain : Gain  Gain=h/tao_m  OutDataTypeStr=fixdt(1,16,8)
  Gain1 : Gain  Gain=Rm
  Gain2 : Gain  Gain=Rm
  HDL Counter : hdlsllib/Sources/HDL Counter  CountType=Count limited  CountInit=0  CountStep=1  CountMax=length(g_lut)-1  CountFromType=Initial value  CountFrom=0  CountResetPort=on  CountLoadPort=off  CountEnbPort=on  CountDirPort=off  CountHitOutputPort=off  CountDataType=Unsigned  CountWordLen=8  CountFracLen=0  CountSampTime=1
  HDL Counter1 : hdlsllib/Sources/HDL Counter  CountType=Count limited  CountInit=0  CountStep=1  CountMax=2  CountFromType=Initial value  CountFrom=0  CountResetPort=off  CountLoadPort=off  CountEnbPort=on  CountDirPort=off  CountHitOutputPort=off  CountDataType=Unsigned  CountWordLen=8  CountFracLen=0  CountSampTime=1
  Logical Operator : Logic  Operator=OR  AllPortsSameDT=off  OutDataTypeStr=boolean
  Logical Operator1 : Logic  Operator=OR  AllPortsSameDT=off  OutDataTypeStr=boolean
  Logical Operator2 : Logic  Operator=OR  AllPortsSameDT=off  OutDataTypeStr=boolean
  Product : Product
  Product1 : Product
  Refractory Counter : hdlsllib/Sources/HDL Counter  CountType=Count limited  CountInit=0  CountStep=1  CountMax=r_time  CountFromType=Initial value  CountFrom=0  CountResetPort=off  CountLoadPort=off  CountEnbPort=on  CountDirPort=off  CountHitOutputPort=off  CountDataType=Unsigned  CountWordLen=8  CountFracLen=0  CountSampTime=1
  Sum of Elements : Sum  Inputs=+
  Sum of Elements1 : Sum  Inputs=+
  Switch : Switch  Criteria=u2 > Threshold  SaturateOnIntegerOverflow=off  InputSameDT=off
  Switch1 : Switch  Criteria=u2 > Threshold  OutDataTypeStr=fixdt(1,16,8)  SaturateOnIntegerOverflow=off  InputSameDT=off
  g : Outport  VectorParamsAs1DForOutWhenUnconnected=off
  wires:
  Constant/1 -> Add2/2
  Delay/1 -> Add3/2, Add4/2, Add/2, Add2/1  "v_past"
  Add/1 -> Switch/3, Compare To Constant/1  "v"
  g_i/1 -> Sum of Elements1/1
  Gain1/1 -> Add1/1
  Add2/1 -> Add1/3
  Add1/1 -> Gain/1
  Add4/1 -> Product1/2
  Product/1 -> Gain1/1
  Add3/1 -> Product/2
  Gain2/1 -> Add1/2
  Gain/1 -> Add/1
  Sum of Elements/1 -> Product/1
  Constant1/1 -> Add3/1
  Constant2/1 -> Add4/1
  Product1/1 -> Gain2/1
  Constant3/1 -> Switch/1
  Refractory Counter/1 -> Logical Operator/2, Switch/2
  Logical Operator/1 -> Refractory Counter/1
  HDL Counter/1 -> Logical Operator1/2, 1-D Lookup Table/1
  Switch1/1 -> g/1
  Switch/1 -> Delay/1
  1-D Lookup Table/1 -> Switch1/3
  Logical Operator1/1 -> HDL Counter/2
  Delay1/1 -> Logical Operator1/1
  Constant4/1 -> Switch1/1
  Logical Operator2/1 -> HDL Counter1/1
  HDL Counter1/1 -> Switch1/2, Logical Operator2/2
  Compare To Constant/1 -> Logical Operator/1, Delay1/1, Logical Operator2/1, HDL Counter/1
  g_e/1 -> Sum of Elements/1
  Sum of Elements1/1 -> Product1/1

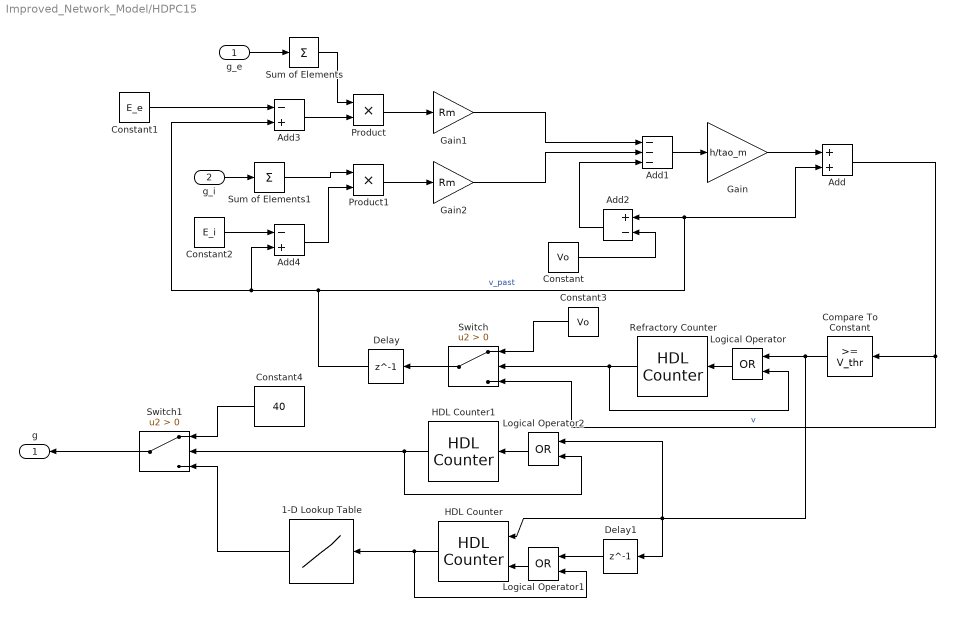
== system Improved_Network_Model/HDPC15 ==
  g_e : Inport
  g_i : Inport  Port=2
  1-D Lookup Table : Lookup_n-D  NumberOfTableDimensions=1  LookupTableObject=''  BreakpointsForDimension1=[0:201]  BreakpointsForDimension1FirstPoint=10  BreakpointsForDimension2FirstPoint=10  BreakpointsForDimension1Spacing=12  BreakpointsForDimension2Spacing=12  BreakpointsForDimension1DataTypeStr=Inherit: Inherit from 'Breakpoint data'  IndexSearchMethod=Evenly spaced points  Table=g_lut  InterpMethod=Flat  DiagnosticForOutOfRangeInput=Error  InternalRulePriority=Speed  OutDataTypeStr=fixdt(1,16,8)  RndMeth=Simplest
  Add : Sum
  Add1 : Sum  Inputs=---
  Add2 : Sum  Inputs=+-
  Add3 : Sum  Inputs=-+
  Add4 : Sum  Inputs=-+
  Compare To Constant : hdlsllib/Logic and Bit Operations/Compare To Constant  relop=>=  const=V_thr  OutDataTypeStr=boolean
  Constant : Constant  Value=Vo  OutDataTypeStr=fixdt(1,16,8)
  Constant1 : Constant  Value=E_e  OutDataTypeStr=fixdt(1,16,8)
  Constant2 : Constant  Value=E_i  OutDataTypeStr=fixdt(1,16,8)
  Constant3 : Constant  Value=Vo  OutDataTypeStr=fixdt(1,16,8)
  Constant4 : Constant  Value=40  OutDataTypeStr=fixdt(1,16,8)
  Delay : Delay  DelayLength=1  InitialCondition=Vo
  Delay1 : Delay  DelayLength=1  InitialCondition=0
  Gain : Gain  Gain=h/tao_m  OutDataTypeStr=fixdt(1,16,8)
  Gain1 : Gain  Gain=Rm
  Gain2 : Gain  Gain=Rm
  HDL Counter : hdlsllib/Sources/HDL Counter  CountType=Count limited  CountInit=0  CountStep=1  CountMax=length(g_lut)-1  CountFromType=Initial value  CountFrom=0  CountResetPort=on  CountLoadPort=off  CountEnbPort=on  CountDirPort=off  CountHitOutputPort=off  CountDataType=Unsigned  CountWordLen=8  CountFracLen=0  CountSampTime=1
  HDL Counter1 : hdlsllib/Sources/HDL Counter  CountType=Count limited  CountInit=0  CountStep=1  CountMax=2  CountFromType=Initial value  CountFrom=0  CountResetPort=off  CountLoadPort=off  CountEnbPort=on  CountDirPort=off  CountHitOutputPort=off  CountDataType=Unsigned  CountWordLen=8  CountFracLen=0  CountSampTime=1
  Logical Operator : Logic  Operator=OR  AllPortsSameDT=off  OutDataTypeStr=boolean
  Logical Operator1 : Logic  Operator=OR  AllPortsSameDT=off  OutDataTypeStr=boolean
  Logical Operator2 : Logic  Operator=OR  AllPortsSameDT=off  OutDataTypeStr=boolean
  Product : Product
  Product1 : Product
  Refractory Counter : hdlsllib/Sources/HDL Counter  CountType=Count limited  CountInit=0  CountStep=1  CountMax=r_time  CountFromType=Initial value  CountFrom=0  CountResetPort=off  CountLoadPort=off  CountEnbPort=on  CountDirPort=off  CountHitOutputPort=off  CountDataType=Unsigned  CountWordLen=8  CountFracLen=0  CountSampTime=1
  Sum of Elements : Sum  Inputs=+
  Sum of Elements1 : Sum  Inputs=+
  Switch : Switch  Criteria=u2 > Threshold  SaturateOnIntegerOverflow=off  InputSameDT=off
  Switch1 : Switch  Criteria=u2 > Threshold  OutDataTypeStr=fixdt(1,16,8)  SaturateOnIntegerOverflow=off  InputSameDT=off
  g : Outport  VectorParamsAs1DForOutWhenUnconnected=off
  wires:
  Constant/1 -> Add2/2
  Delay/1 -> Add3/2, Add4/2, Add/2, Add2/1  "v_past"
  Add/1 -> Switch/3, Compare To Constant/1  "v"
  g_i/1 -> Sum of Elements1/1
  Gain1/1 -> Add1/1
  Add2/1 -> Add1/3
  Add1/1 -> Gain/1
  Add4/1 -> Product1/2
  Product/1 -> Gain1/1
  Add3/1 -> Product/2
  Gain2/1 -> Add1/2
  Gain/1 -> Add/1
  Sum of Elements/1 -> Product/1
  Constant1/1 -> Add3/1
  Constant2/1 -> Add4/1
  Product1/1 -> Gain2/1
  Constant3/1 -> Switch/1
  Refractory Counter/1 -> Logical Operator/2, Switch/2
  Logical Operator/1 -> Refractory Counter/1
  HDL Counter/1 -> Logical Operator1/2, 1-D Lookup Table/1
  Switch1/1 -> g/1
  Switch/1 -> Delay/1
  1-D Lookup Table/1 -> Switch1/3
  Logical Operator1/1 -> HDL Counter/2
  Delay1/1 -> Logical Operator1/1
  Constant4/1 -> Switch1/1
  Logical Operator2/1 -> HDL Counter1/1
  HDL Counter1/1 -> Switch1/2, Logical Operator2/2
  Compare To Constant/1 -> Logical Operator/1, Delay1/1, Logical Operator2/1, HDL Counter/1
  g_e/1 -> Sum of Elements/1
  Sum of Elements1/1 -> Product1/1

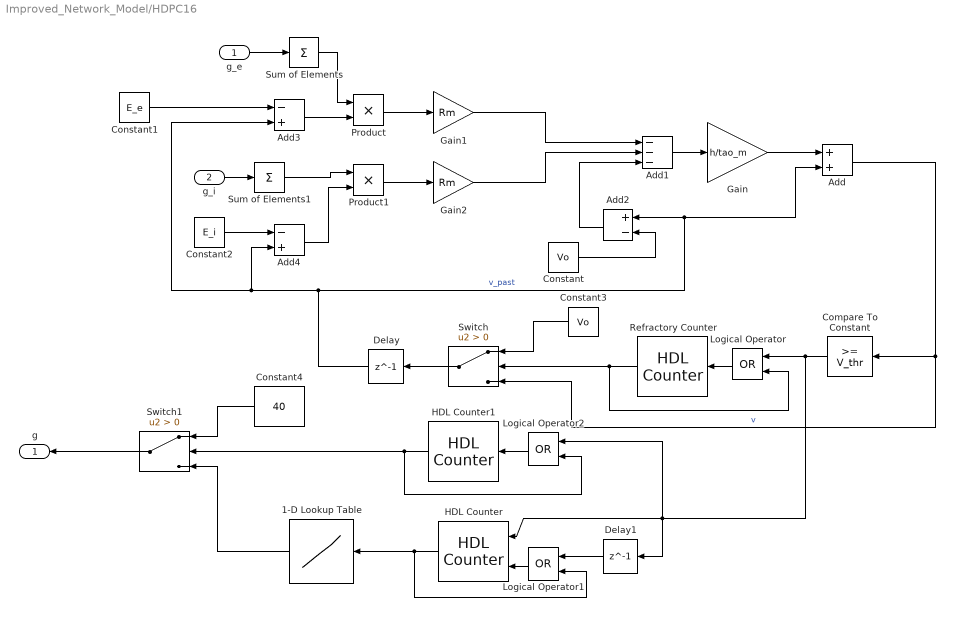
== system Improved_Network_Model/HDPC16 ==
  g_e : Inport
  g_i : Inport  Port=2
  1-D Lookup Table : Lookup_n-D  NumberOfTableDimensions=1  LookupTableObject=''  BreakpointsForDimension1=[0:201]  BreakpointsForDimension1FirstPoint=10  BreakpointsForDimension2FirstPoint=10  BreakpointsForDimension1Spacing=12  BreakpointsForDimension2Spacing=12  BreakpointsForDimension1DataTypeStr=Inherit: Inherit from 'Breakpoint data'  IndexSearchMethod=Evenly spaced points  Table=g_lut  InterpMethod=Flat  DiagnosticForOutOfRangeInput=Error  InternalRulePriority=Speed  OutDataTypeStr=fixdt(1,16,8)  RndMeth=Simplest
  Add : Sum
  Add1 : Sum  Inputs=---
  Add2 : Sum  Inputs=+-
  Add3 : Sum  Inputs=-+
  Add4 : Sum  Inputs=-+
  Compare To Constant : hdlsllib/Logic and Bit Operations/Compare To Constant  relop=>=  const=V_thr  OutDataTypeStr=boolean
  Constant : Constant  Value=Vo  OutDataTypeStr=fixdt(1,16,8)
  Constant1 : Constant  Value=E_e  OutDataTypeStr=fixdt(1,16,8)
  Constant2 : Constant  Value=E_i  OutDataTypeStr=fixdt(1,16,8)
  Constant3 : Constant  Value=Vo  OutDataTypeStr=fixdt(1,16,8)
  Constant4 : Constant  Value=40  OutDataTypeStr=fixdt(1,16,8)
  Delay : Delay  DelayLength=1  InitialCondition=Vo
  Delay1 : Delay  DelayLength=1  InitialCondition=0
  Gain : Gain  Gain=h/tao_m  OutDataTypeStr=fixdt(1,16,8)
  Gain1 : Gain  Gain=Rm
  Gain2 : Gain  Gain=Rm
  HDL Counter : hdlsllib/Sources/HDL Counter  CountType=Count limited  CountInit=0  CountStep=1  CountMax=length(g_lut)-1  CountFromType=Initial value  CountFrom=0  CountResetPort=on  CountLoadPort=off  CountEnbPort=on  CountDirPort=off  CountHitOutputPort=off  CountDataType=Unsigned  CountWordLen=8  CountFracLen=0  CountSampTime=1
  HDL Counter1 : hdlsllib/Sources/HDL Counter  CountType=Count limited  CountInit=0  CountStep=1  CountMax=2  CountFromType=Initial value  CountFrom=0  CountResetPort=off  CountLoadPort=off  CountEnbPort=on  CountDirPort=off  CountHitOutputPort=off  CountDataType=Unsigned  CountWordLen=8  CountFracLen=0  CountSampTime=1
  Logical Operator : Logic  Operator=OR  AllPortsSameDT=off  OutDataTypeStr=boolean
  Logical Operator1 : Logic  Operator=OR  AllPortsSameDT=off  OutDataTypeStr=boolean
  Logical Operator2 : Logic  Operator=OR  AllPortsSameDT=off  OutDataTypeStr=boolean
  Product : Product
  Product1 : Product
  Refractory Counter : hdlsllib/Sources/HDL Counter  CountType=Count limited  CountInit=0  CountStep=1  CountMax=r_time  CountFromType=Initial value  CountFrom=0  CountResetPort=off  CountLoadPort=off  CountEnbPort=on  CountDirPort=off  CountHitOutputPort=off  CountDataType=Unsigned  CountWordLen=8  CountFracLen=0  CountSampTime=1
  Sum of Elements : Sum  Inputs=+
  Sum of Elements1 : Sum  Inputs=+
  Switch : Switch  Criteria=u2 > Threshold  SaturateOnIntegerOverflow=off  InputSameDT=off
  Switch1 : Switch  Criteria=u2 > Threshold  OutDataTypeStr=fixdt(1,16,8)  SaturateOnIntegerOverflow=off  InputSameDT=off
  g : Outport  VectorParamsAs1DForOutWhenUnconnected=off
  wires:
  Constant/1 -> Add2/2
  Delay/1 -> Add3/2, Add4/2, Add/2, Add2/1  "v_past"
  Add/1 -> Switch/3, Compare To Constant/1  "v"
  g_i/1 -> Sum of Elements1/1
  Gain1/1 -> Add1/1
  Add2/1 -> Add1/3
  Add1/1 -> Gain/1
  Add4/1 -> Product1/2
  Product/1 -> Gain1/1
  Add3/1 -> Product/2
  Gain2/1 -> Add1/2
  Gain/1 -> Add/1
  Sum of Elements/1 -> Product/1
  Constant1/1 -> Add3/1
  Constant2/1 -> Add4/1
  Product1/1 -> Gain2/1
  Constant3/1 -> Switch/1
  Refractory Counter/1 -> Logical Operator/2, Switch/2
  Logical Operator/1 -> Refractory Counter/1
  HDL Counter/1 -> Logical Operator1/2, 1-D Lookup Table/1
  Switch1/1 -> g/1
  Switch/1 -> Delay/1
  1-D Lookup Table/1 -> Switch1/3
  Logical Operator1/1 -> HDL Counter/2
  Delay1/1 -> Logical Operator1/1
  Constant4/1 -> Switch1/1
  Logical Operator2/1 -> HDL Counter1/1
  HDL Counter1/1 -> Switch1/2, Logical Operator2/2
  Compare To Constant/1 -> Logical Operator/1, Delay1/1, Logical Operator2/1, HDL Counter/1
  g_e/1 -> Sum of Elements/1
  Sum of Elements1/1 -> Product1/1

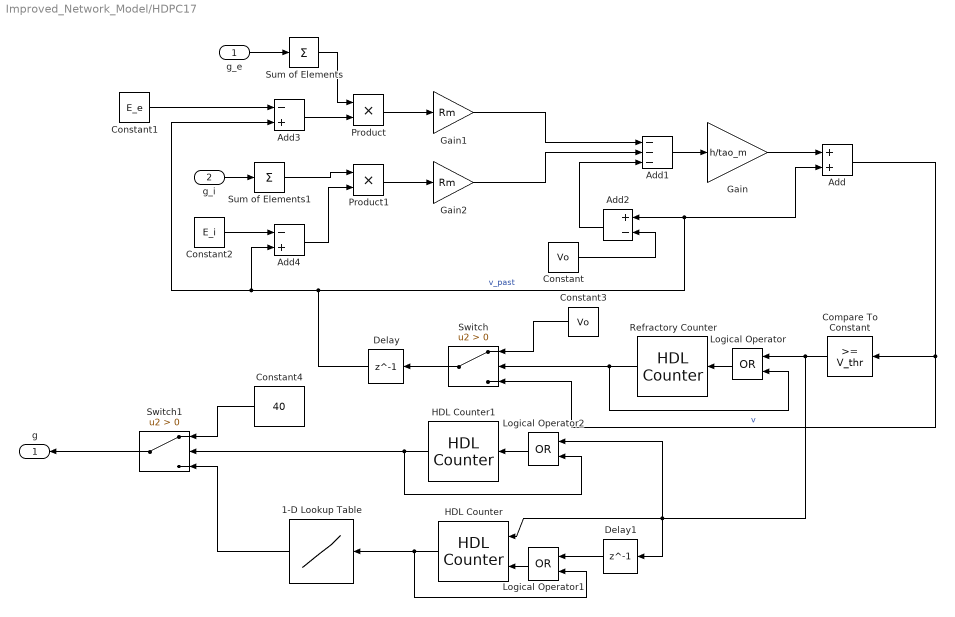
== system Improved_Network_Model/HDPC17 ==
  g_e : Inport
  g_i : Inport  Port=2
  1-D Lookup Table : Lookup_n-D  NumberOfTableDimensions=1  LookupTableObject=''  BreakpointsForDimension1=[0:201]  BreakpointsForDimension1FirstPoint=10  BreakpointsForDimension2FirstPoint=10  BreakpointsForDimension1Spacing=12  BreakpointsForDimension2Spacing=12  BreakpointsForDimension1DataTypeStr=Inherit: Inherit from 'Breakpoint data'  IndexSearchMethod=Evenly spaced points  Table=g_lut  InterpMethod=Flat  DiagnosticForOutOfRangeInput=Error  InternalRulePriority=Speed  OutDataTypeStr=fixdt(1,16,8)  RndMeth=Simplest
  Add : Sum
  Add1 : Sum  Inputs=---
  Add2 : Sum  Inputs=+-
  Add3 : Sum  Inputs=-+
  Add4 : Sum  Inputs=-+
  Compare To Constant : hdlsllib/Logic and Bit Operations/Compare To Constant  relop=>=  const=V_thr  OutDataTypeStr=boolean
  Constant : Constant  Value=Vo  OutDataTypeStr=fixdt(1,16,8)
  Constant1 : Constant  Value=E_e  OutDataTypeStr=fixdt(1,16,8)
  Constant2 : Constant  Value=E_i  OutDataTypeStr=fixdt(1,16,8)
  Constant3 : Constant  Value=Vo  OutDataTypeStr=fixdt(1,16,8)
  Constant4 : Constant  Value=40  OutDataTypeStr=fixdt(1,16,8)
  Delay : Delay  DelayLength=1  InitialCondition=Vo
  Delay1 : Delay  DelayLength=1  InitialCondition=0
  Gain : Gain  Gain=h/tao_m  OutDataTypeStr=fixdt(1,16,8)
  Gain1 : Gain  Gain=Rm
  Gain2 : Gain  Gain=Rm
  HDL Counter : hdlsllib/Sources/HDL Counter  CountType=Count limited  CountInit=0  CountStep=1  CountMax=length(g_lut)-1  CountFromType=Initial value  CountFrom=0  CountResetPort=on  CountLoadPort=off  CountEnbPort=on  CountDirPort=off  CountHitOutputPort=off  CountDataType=Unsigned  CountWordLen=8  CountFracLen=0  CountSampTime=1
  HDL Counter1 : hdlsllib/Sources/HDL Counter  CountType=Count limited  CountInit=0  CountStep=1  CountMax=2  CountFromType=Initial value  CountFrom=0  CountResetPort=off  CountLoadPort=off  CountEnbPort=on  CountDirPort=off  CountHitOutputPort=off  CountDataType=Unsigned  CountWordLen=8  CountFracLen=0  CountSampTime=1
  Logical Operator : Logic  Operator=OR  AllPortsSameDT=off  OutDataTypeStr=boolean
  Logical Operator1 : Logic  Operator=OR  AllPortsSameDT=off  OutDataTypeStr=boolean
  Logical Operator2 : Logic  Operator=OR  AllPortsSameDT=off  OutDataTypeStr=boolean
  Product : Product
  Product1 : Product
  Refractory Counter : hdlsllib/Sources/HDL Counter  CountType=Count limited  CountInit=0  CountStep=1  CountMax=r_time  CountFromType=Initial value  CountFrom=0  CountResetPort=off  CountLoadPort=off  CountEnbPort=on  CountDirPort=off  CountHitOutputPort=off  CountDataType=Unsigned  CountWordLen=8  CountFracLen=0  CountSampTime=1
  Sum of Elements : Sum  Inputs=+
  Sum of Elements1 : Sum  Inputs=+
  Switch : Switch  Criteria=u2 > Threshold  SaturateOnIntegerOverflow=off  InputSameDT=off
  Switch1 : Switch  Criteria=u2 > Threshold  OutDataTypeStr=fixdt(1,16,8)  SaturateOnIntegerOverflow=off  InputSameDT=off
  g : Outport  VectorParamsAs1DForOutWhenUnconnected=off
  wires:
  Constant/1 -> Add2/2
  Delay/1 -> Add3/2, Add4/2, Add/2, Add2/1  "v_past"
  Add/1 -> Switch/3, Compare To Constant/1  "v"
  g_i/1 -> Sum of Elements1/1
  Gain1/1 -> Add1/1
  Add2/1 -> Add1/3
  Add1/1 -> Gain/1
  Add4/1 -> Product1/2
  Product/1 -> Gain1/1
  Add3/1 -> Product/2
  Gain2/1 -> Add1/2
  Gain/1 -> Add/1
  Sum of Elements/1 -> Product/1
  Constant1/1 -> Add3/1
  Constant2/1 -> Add4/1
  Product1/1 -> Gain2/1
  Constant3/1 -> Switch/1
  Refractory Counter/1 -> Logical Operator/2, Switch/2
  Logical Operator/1 -> Refractory Counter/1
  HDL Counter/1 -> Logical Operator1/2, 1-D Lookup Table/1
  Switch1/1 -> g/1
  Switch/1 -> Delay/1
  1-D Lookup Table/1 -> Switch1/3
  Logical Operator1/1 -> HDL Counter/2
  Delay1/1 -> Logical Operator1/1
  Constant4/1 -> Switch1/1
  Logical Operator2/1 -> HDL Counter1/1
  HDL Counter1/1 -> Switch1/2, Logical Operator2/2
  Compare To Constant/1 -> Logical Operator/1, Delay1/1, Logical Operator2/1, HDL Counter/1
  g_e/1 -> Sum of Elements/1
  Sum of Elements1/1 -> Product1/1
